simulink model "Half_Bridge_Inverter"  (R2014a)
settings: Solver=ode45  StartTime=0.0  StopTime=0.05  RelTol=1e-3
libraries: powerlib x8
settings Model: Creator=RAVINDERNATH YADAV  LastModifiedBy=RAVINDERNATH YADAV

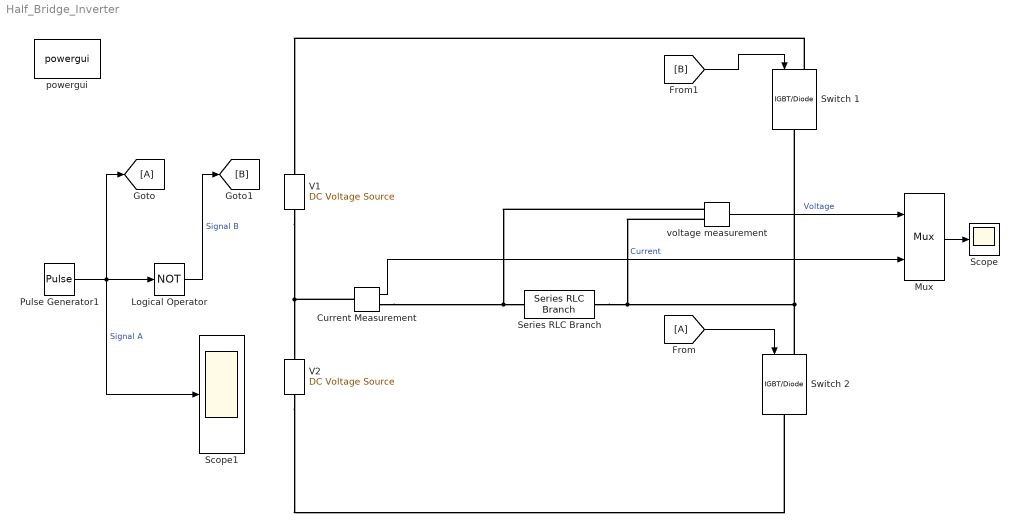
== system Half_Bridge_Inverter ==
  Current Measurement : powerlib/Measurements/Current Measurement  PhasorSimulation=off  OutputType=Complex  PSBequivalent=0
  Logical Operator : Logic  Operator=NOT  AllPortsSameDT=off  OutDataTypeStr=boolean
  Mux : Mux  Inputs=2
  Pulse Generator1 : DiscretePulseGenerator  PulseType=Time based  Period=0.01  PulseWidth=50
  Scope : Scope
      settings: TickLabels=on  ShowLegends=on  YMin=-3  YMax=3
  Scope1 : Scope
      settings: TickLabels=on  ShowLegends=on  YMin=-0.1  YMax=1.5
  Series RLC Branch : powerlib/Elements/Series RLC Branch  LConnTagsString=__new0  RConnTagsString=__new0  BranchType=R  Resistance=10  Inductance=1e-3  SetiL0=off  InitialCurrent=0  Capacitance=1e-6  Setx0=off  InitialVoltage=0  Measurements=None
  Switch 1 : powerlib/Power Electronics/IGBT//Diode  Ron=1e-3  Rs=1e5  Cs=inf  Measurements=off
  Switch 2 : powerlib/Power Electronics/IGBT//Diode  Ron=1e-3  Rs=1e5  Cs=inf  Measurements=off
  V1 : powerlib/Electrical Sources/DC Voltage Source  Amplitude=2  Measurements=Voltage
  V2 : powerlib/Electrical Sources/DC Voltage Source  Amplitude=2  Measurements=Voltage
  powergui : powerlib/powergui  Priority=1  SimulationMode=Discrete  SolverType=Tustin  SampleTime=50e-6  frequency=60  SPID=off  DisableSnubberDevices=off  DisableRonSwitches=off  DisableVfSwitches=off  SwTol=0  Interpol=off  DisplayEquations=off  Ts=0  methode=off  frequencyindice=0  Pbase=100e6  ErrMax=1e-4  Iterations=50  UnitsV=kV  UnitsW=MW  FunctionMessages=off  echomessages=off  HookPort=off  EnableUseOfTLC=off  x0status=blocks  RestoreLinks=warning  ResistiveCurrentMeasurement=off  Frange=[0:2:500]  Ylog=off  Xlog=on  ShowGrid=off  save=off  variable=ZData  structure=0  ZoomFFT=off  StartTime=0.0  cycles=1  DisplayStyle=1  fundamental=60  FreqAxis=off  MaxFrequency=1000  frequencyindicesteady=1  RmsSteady=1  display=off
  "voltage measurement " : powerlib/Measurements/Voltage Measurement  PhasorSimulation=off  OutputType=Complex  PSBequivalent=0
  wires:
  Pulse Generator1/1 -> Scope1/1, [A], Logical Operator/1  "Signal A"
  [B] -> Switch 1/1
  Logical Operator/1 -> [B]  "Signal B"
  [A] -> Switch 2/1
  Current Measurement/1 -> Mux/2  "Current"
  "voltage measurement "/1 -> Mux/1  "Voltage"
  Mux/1 -> Scope/1
  connections:
  V1/LConn1 -- V2/RConn1 -- Current Measurement/LConn1
  Current Measurement/RConn1 -- "voltage measurement "/LConn1 -- Series RLC Branch/LConn1
  Series RLC Branch/RConn1 -- "voltage measurement "/LConn2 -- Switch 2/LConn1 -- Switch 1/RConn1
  Switch 1/LConn1 -- V1/RConn1
  V2/LConn1 -- Switch 2/RConn1
